simulink model "MPC_simulation"  (R2020a)
settings: Solver=VariableStepAuto  StartTime=0.0  StopTime=100  RelTol=1e-3
values from neighbouring files (symbols this model uses):
  Q = u(6)    [MPC_controller.m]
  R = u(7)    [MPC_controller.m]
undefined symbols (not defined in the file or in its folder): A, B, C, G, H, Np, Ts
settings Model: Creator=Huiqian  LastModifiedBy=Huiqian

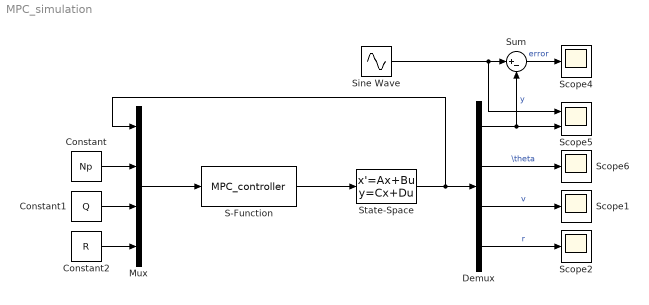
== system MPC_simulation ==
  Constant : Constant  Value=Np
  Constant1 : Constant  Value=Q
  Constant2 : Constant  Value=R
  Demux : Demux
  Mux : Mux  Inputs=[4,1,1,1]
  S-Function : S-Function  FunctionName=MPC_controller  Parameters=G,H,Ts  SFunctionDeploymentMode=off  EnableBusSupport=off
  Scope{1..2,4,6} (4 alike) : Scope
  Scope5 : Scope  NumInputPorts=2
  Sine Wave : Sin  Amplitude=2  Frequency=0.1*pi  SampleTime=0
  State-Space : StateSpace  A=A  B=B  C=C  D=zeros(size(C,1),1)  InitialCondition=0
  Sum : Sum  Inputs=|+-
  wires:
  S-Function/1 -> State-Space/1
  State-Space/1 -> Mux/1, Demux/1
  Demux/1 -> Scope5/2, Sum/2  "y"
  Demux/2 -> Scope6/1  "\\theta"
  Demux/3 -> Scope1/1  "v"
  Demux/4 -> Scope2/1  "r"
  Sine Wave/1 -> Scope5/1, Sum/1
  Sum/1 -> Scope4/1  "error"
  Mux/1 -> S-Function/1
  Constant/1 -> Mux/2
  Constant1/1 -> Mux/3
  Constant2/1 -> Mux/4
